simulink model "mod1_delint"  (Simulink 8.1)
settings: Solver=FixedStepDiscrete  StartTime=0.0  StopTime=10e-3  RelTol=1e-3
undefined symbols (not defined in the file): modctrl
libraries: dspsigops x1, dspsrcs4 x1
settings Model: Creator=amyles  LastModifiedBy=amyles
settings DataIOCC: LimitDataPoints=off  MaxDataPoints=50000
settings OptimizationCC: InlineParams=on
settings DebuggingCC: StrictBusMsg=Warning
settings ModelReferenceCC: ModelReferenceNumInstancesAllowed=Single

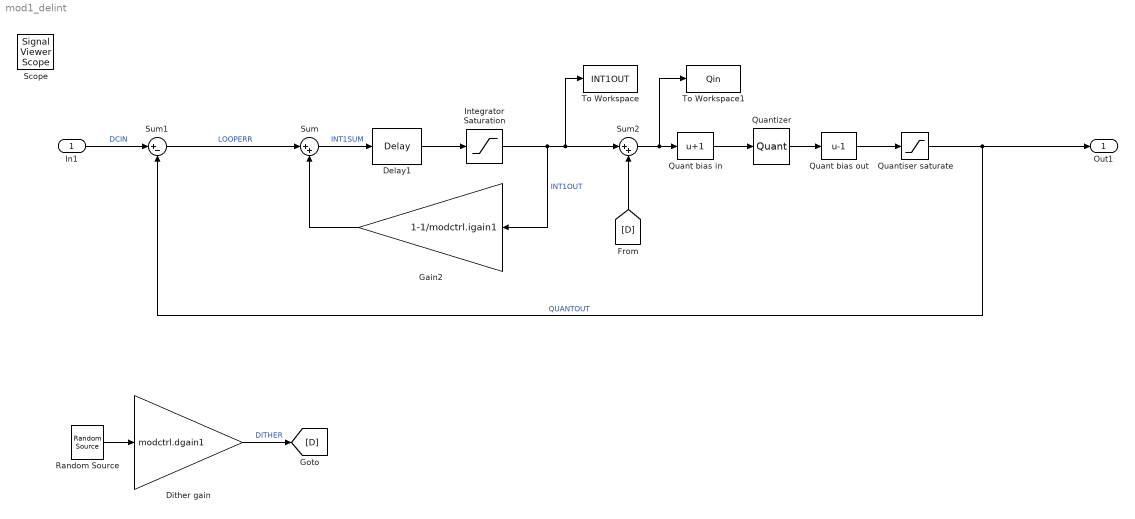
== system mod1_delint ==
  In1 : Inport
  Delay1 : dspsigops/Delay  InputProcessing=Inherited (this choice will be removed - see release notes)  dly_unit=Samples  delay=1  ic_detail=off  dif_ic_for_ch=off  dif_ic_for_dly=off  ic=0  reset_popup=None
  Dither gain : Gain  Gain=modctrl.dgain1
      settings: AttributesFormatString=Dither level adjust
  Gain2 : Gain  Gain=1-1/modctrl.igain1
      settings: AttributesFormatString=(model finite dc gain)
  Integrator Saturation : Saturate  UpperLimit=modctrl.isat1  LowerLimit=-(modctrl.isat1)
  Quant bias in : Bias  Bias=1
      settings: AttributesFormatString=Need offset to give\nMID-RISE quantiser
  Quant bias out : Bias  Bias=-1
      settings: AttributesFormatString=Shift outputs to\n..., -2, 1, 1, ...
  Quantiser saturate : Saturate  UpperLimit=1  LowerLimit=-1
      settings: AttributesFormatString=Limit quantiser\noutput to +/-1
  Quantizer : Quantizer  QuantizationInterval=2  LinearizeAsGain=off
      settings: AttributesFormatString=step = 2
  Random Source : dspsrcs4/Random Source  SrcType=Uniform  NormMethod=Ziggurat  CltLength=12  MinVal=-1  MaxVal=1  MeanVal=0  VarVal=1  RepMode=Not repeatable  rawSeed=1  IsInherit=off  SampMode=Discrete  SampTime=1e-6  SampFrame=1  DataType=Double  OutComplex=Real
      settings: AttributesFormatString=Dither source
  Sum : Sum  Inputs=|++
      settings: AttributesFormatString=Integrator summer
  Sum1 : Sum  Inputs=|+-
      settings: AttributesFormatString=Modulator input\nloop servo error (input - fbk)
  Sum2 : Sum  Inputs=|++
  To Workspace : ToWorkspace  VariableName=INT1OUT  SampleTime=-1  SaveFormat=Structure
  To Workspace1 : ToWorkspace  VariableName=Qin  SampleTime=-1  SaveFormat=Structure
  Out1 : Outport
  Scope : SignalViewerScope  IOType=viewer  NumInputPorts=2  ZoomMode=xonly  RefreshTime=0.035000
      settings: YMin=-5~-5  YMax=5~5
  wires:
  Sum/1 -> Delay1/1  "INT1SUM"
  Sum1/1 -> Sum/1  "LOOPERR"
  In1/1 -> Sum1/1  "DCIN"
  Random Source/1 -> Dither gain/1
  Gain2/1 -> Sum/2
  Integrator Saturation/1 -> Gain2/1, Sum2/1, To Workspace/1  "INT1OUT"
  Delay1/1 -> Integrator Saturation/1
  Dither gain/1 -> [D]  "DITHER"
  [D] -> Sum2/2
  Sum2/1 -> Quant bias in/1, To Workspace1/1
  Quantiser saturate/1 -> Out1/1, Sum1/2  "QUANTOUT"
  Quant bias out/1 -> Quantiser saturate/1
  Quantizer/1 -> Quant bias out/1
  Quant bias in/1 -> Quantizer/1
